simulink model "Core_Model"  (R2023a)
settings: Solver=FixedStepAuto  StartTime=0  StopTime=Z  FixedStep=1/24  RelTol=1e-3
values from neighbouring files (symbols this model uses):
  c_eh = 0.85    [Model_Parameters.m]
  cc_e = -0.85    [Model_Parameters.m]
  R_H2 = 0.05    [Model_Parameters.m]
  R_lh = 0.025    [Model_Parameters.m]
  R_ng = 0.025    [Model_Parameters.m]
libraries: fl_lib x63, nesl_utility x48, ee_lib x22
(part 2 of 2)

== matlab function Core_Model/Seasonal ==
  data: X input; wind_distr output
function wind_distr= fcn(X)

%% Parameters
a0 = 9.564;
a1 = 1.636;
b1 = 0.4314;
a2 = 0.2612;
b2 = 0.2799;
a3 = -0.4869;
b3 = 0.4023;
a4 = -0.141;
b4 = 0.06985;
a5 = 0.1669;
b5 = 0.03972;
w = 0.01721;

% % c0 = 9.839;
% c1 = 0.2685;
% d1 = -0.1482;
% c2 = -0.08017;
% d2 = -0.08146;
% w2 = 6.288;


       aa0 =       10.21  ;
       aa1 =      0.1631 ;
       bb1 =     -0.2515 ;
       aa2 =    -0.05622  ;
       bb2 =    -0.08132  ;
       aa3 =    -0.01446  ;
       bb3 =     0.01009  ;
       ww =      6.545;
%% Generate wind distributions
yearly_w = a0 + a1*cos(X*w) + b1*sin(X*w) + a2*cos(2*X*w) + b2*sin(2*X*w) + a3*cos(3*X*w) + b3*sin(3*X*w) + a4*cos(4*X*w) + b4*sin(4*X*w) + a5*cos(5*X*w) + b5*sin(5*X*w);
% daily_w = c1*cos(X*w2) + d1*sin(X*w2) + c2*cos(2*X*w2) + d2*sin(2*X*w2);


% Convert X from days to hours by dividing by 24
X_in_hours = X ;

daily_w =  aa1*cos(X_in_hours*ww) + bb1*sin(X_in_hours*ww) + aa2*cos(2*X_in_hours*ww) + bb2*sin(2*X_in_hours*ww) + aa3*cos(3*X_in_hours*ww) + bb3*sin(3*X_in_hours*ww);
    

% Total wind distribution
wind_distr = yearly_w + daily_w; %TNO: Offshore wind energy deployment in the North Sea by 2030: long-term measurement campaign.EPL, 2016-2020

end

== matlab function Core_Model/OWE gen ==
  data: wind_distr input; current output
function current= fcn(wind_distr)
wind=wind_distr;

%% Wind to Electricity

       
    % Power curve
    wind_speeds = [0, 2, 4, 6, 8, 10, 12, 14, 16, 18, 20, 22, 24, 26]; % Wind speed values
    power_output = [0, 0, 0.5, 1, 3.7, 4.7, 6.3, 9.5, 9.5, 9.5, 9.5, 9.5, 0, 0]; % Corresponding power output values  in MW
    %powercurve: https://www.researchgate.net/figure/Power-curve-of-the-Vestas-V164-95-turbine-including-some-technical-data-left-side-and_fig4_351600993

    % Interpolate the power curve
    power_curve = interp1(wind_speeds, power_output, wind, 'linear', 'extrap');  % 'extrap' for extrapolation MW/turbine = MW/9.5MW
    
    % Limit power output to positive values
    power_curve(power_curve < 0) = 0;

    % Apply the power curve to wind speed samples
    electricity_production = power_curve .* wind; %MW

    % Consider turbine availability and capacity if applicable
    availability_factor = 1; % Availability factor
    offshore_wind_capacity = 12e3; % Offshore wind capacity in MW (=10GW)
    nr_turbines=offshore_wind_capacity/9.5;
    % offshore_wind_capacity = 30; % Offshore wind capacity in MW

    % Produced electricity
    electricity_production_MW = electricity_production * availability_factor * nr_turbines; %MWh
    electricity_production_GW = electricity_production_MW*1e-3;

    %% Scaling to integrate within the model 
    % current = 2e7 * electricity_production;
    current = electricity_production_GW/26^2; %GWh/h

    % \ 0.0002*30/10*0.5
end
